simulink model "BSP_v1"  (R2024b)
settings: Solver=VariableStepAuto  StartTime=0.0  StopTime=10.0  RelTol=1e-3
settings Model: Creator=satyendra  LastModifiedBy=satyendra

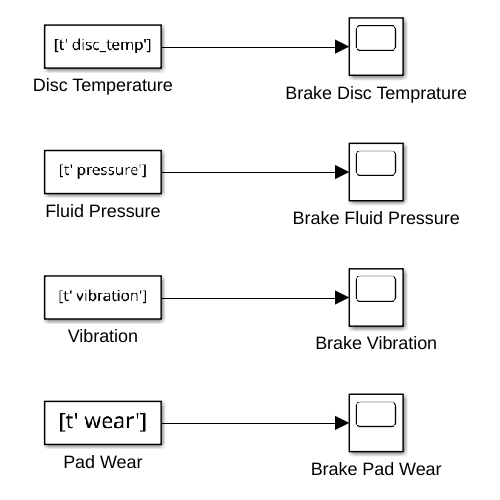
[thumbnail: Simulink's stored preview of the top-level diagram]
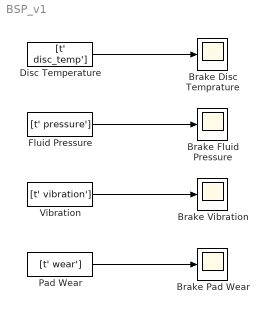
== system BSP_v1 ==
  Brake Disc Temprature : Scope
  Brake Fluid Pressure : Scope
  Brake Pad Wear : Scope
  Brake Vibration : Scope
  Disc Temperature : FromWorkspace  VariableName=[t' disc_temp']
  Fluid Pressure : FromWorkspace  VariableName=[t' pressure']
  Pad Wear : FromWorkspace  VariableName=[t' wear']
  Vibration : FromWorkspace  VariableName=[t' vibration']
  wires:
  Disc Temperature/1 -> Brake Disc Temprature/1
  Fluid Pressure/1 -> Brake Fluid Pressure/1
  Vibration/1 -> Brake Vibration/1
  Pad Wear/1 -> Brake Pad Wear/1
